simulink model "optper"  (Simulink 3.00)
settings: Solver=ode45  SolverMode=SingleTasking  StartTime=0.0  StopTime=250  RelTol=1e-5  AbsTol=1e-5
libraries: simulink_extras x1
settings Model: SaveTime=off  SaveOutput=off  RTWTemplateMakefile=grt_vc.tmf  LastModifiedBy=abonyij

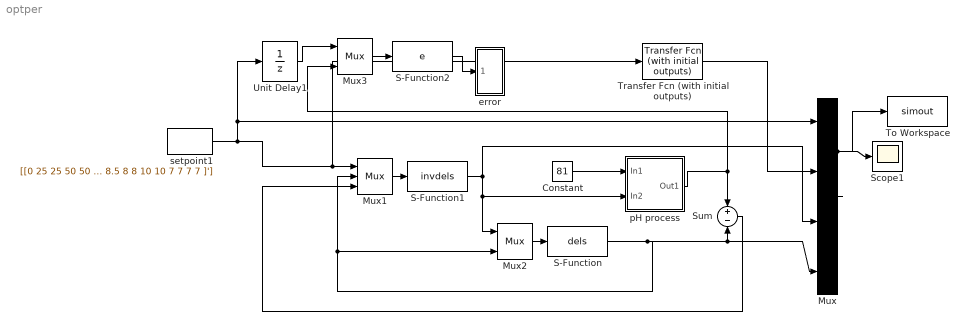
== system optper ==
  Constant : Constant  Value=81
  Mux : Mux  Inputs=4
      settings: DisplayOption=none
  Mux1 : Mux  Inputs=3
      settings: DisplayOption=none
  Mux2 : Mux  Inputs=2
      settings: DisplayOption=none
  Mux3 : Mux  Inputs=2
      settings: DisplayOption=none
  S-Function : S-Function  FunctionName=dels  PortCounts=[]  SFunctionModules=''
  S-Function1 : S-Function  FunctionName=invdels  PortCounts=[]  SFunctionModules=''
  S-Function2 : S-Function  FunctionName=e  PortCounts=[]  SFunctionModules=''
  Scope1 : Scope
      settings: TickLabels=on  TimeRange=auto  YMin=6  YMax=12  SaveName=pi  DataFormat=Matrix  SampleInput=on
  Sum : Sum  Inputs=+|-  SaturateOnIntegerOverflow=on
  To Workspace : ToWorkspace  VariableName=simout  SampleTime=0.2  SaveFormat=Matrix
  Transfer Fcn (with initial outputs) : simulink_extras/Additional Linear/Transfer Fcn (with initial outputs)  N=[1]  D=[0.2 1]  Y0=7  U0=7
  Unit Delay1 : UnitDelay  X0=7  SampleTime=0.2
  error : Subsystem
      mask Display: disp('IAE')
  pH process : Subsystem
  setpoint1 : FromWorkspace  VariableName=[[0 25 25 50 50 75 75 100 100 125 125 150 150 175 175 200 200 225 225 250 250]', [7 8 8 9 9 8 8 9.5 9.4 7.5 7.5 8.5 8.5 8 8 10 10 7 7 7 7 ]']  SampleTime=25  HoldFinalValue=on
  wires:
  Mux/1 -> Scope1/1, To Workspace/1
  Constant/1 -> pH process/1(In1)
  Mux2/1 -> S-Function/1
  Mux1/1 -> S-Function1/1
  S-Function1/1 -> Mux/3, pH process/2(In2), Mux2/1
  S-Function/1 -> Mux/4, Sum/2, Mux1/2, Mux2/2
  Sum/1 -> Mux1/3
  setpoint1/1 -> Mux/1, Unit Delay1/1, Mux1/1, Transfer Fcn (with initial outputs)/1
  S-Function2/1 -> error/1(in_1)
  Mux3/1 -> S-Function2/1
  Unit Delay1/1 -> Mux3/1
  pH process/1(Out1) -> Sum/1, Mux3/2
  Transfer Fcn (with initial outputs)/1 -> Mux/2

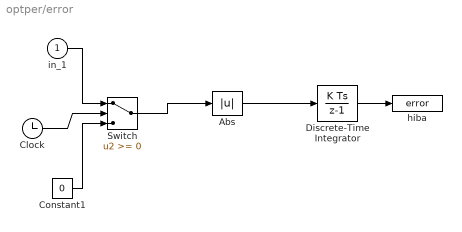
== system optper/error ==
  in_1 : Inport  Port=1  PortWidth=-1  SampleTime=-1  DataType=auto
      settings: SignalType=auto
  Abs : Abs
  Clock : Clock
      settings: DisplayTime=off  Decimation=10
  Constant1 : Constant  Value=0
  Discrete-Time Integrator : DiscreteIntegrator  IntegratorMethod=ForwardEuler  ExternalReset=none  InitialConditionSource=internal  InitialCondition=0  LimitOutput=off  UpperSaturationLimit=inf  LowerSaturationLimit=-inf  ShowSaturationPort=off  ShowStatePort=off  SampleTime=0.2
  Switch : Switch  Threshold=0
  hiba : ToWorkspace  VariableName=error  SampleTime=0  SaveFormat=Matrix
      settings: Buffer=1
  wires:
  Switch/1 -> Abs/1
  in_1/1 -> Switch/1
  Constant1/1 -> Switch/3
  Clock/1 -> Switch/2
  Abs/1 -> Discrete-Time Integrator/1
  Discrete-Time Integrator/1 -> hiba/1

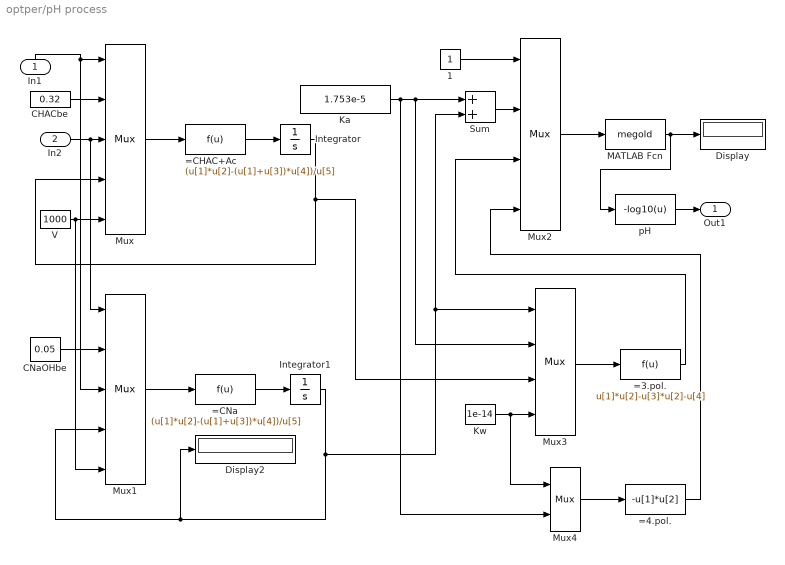
== system optper/pH process ==
  In1 : Inport  Orientation=up  Port=1  PortWidth=-1  SampleTime=-1  DataType=auto
      settings: SignalType=auto
  In2 : Inport  Port=2  PortWidth=-1  SampleTime=-1  DataType=auto
      settings: SignalType=auto
  1 : Constant  Value=1
  =3.pol. : Fcn  Expr=u[1]*u[2]-u[3]*u[2]-u[4]
  =4.pol. : Fcn  Expr=-u[1]*u[2]
  =CHAC+Ac : Fcn  Expr=(u[1]*u[2]-(u[1]+u[3])*u[4])/u[5]
  =CNa : Fcn  Expr=(u[1]*u[2]-(u[1]+u[3])*u[4])/u[5]
  CHACbe : Constant  Value=0.32
  CNaOHbe : Constant  Value=0.05
  Display : Display
      settings: Format=short
  Display2 : Display
      settings: Format=short
  Integrator : Integrator  ExternalReset=none  InitialConditionSource=internal  InitialCondition=0.0435  LimitOutput=off  UpperSaturationLimit=inf  LowerSaturationLimit=-inf  ShowSaturationPort=off  ShowStatePort=off  AbsoluteTolerance=auto
  Integrator1 : Integrator  ExternalReset=none  InitialConditionSource=internal  InitialCondition=0.0432  LimitOutput=off  UpperSaturationLimit=inf  LowerSaturationLimit=-inf  ShowSaturationPort=off  ShowStatePort=off  AbsoluteTolerance=auto
  Ka : Constant  Value=1.753e-5
  Kw : Constant  Value=1e-14
  MATLAB Fcn : MATLABFcn  MATLABFcn=megold  OutputWidth=1  OutputSignalType=auto
  Mux : Mux  Inputs=5
      settings: DisplayOption=none
  Mux1 : Mux  Inputs=5
      settings: DisplayOption=none
  Mux2 : Mux  Inputs=4
      settings: DisplayOption=none
  Mux3 : Mux  Inputs=4
      settings: DisplayOption=none
  Mux4 : Mux  Inputs=2
      settings: DisplayOption=none
  Sum : Sum  Inputs=++  SaturateOnIntegerOverflow=on
  V : Constant  Value=1000
  pH : Fcn  Expr=-log10(u)
  Out1 : Outport  Port=1  InitialOutput=0
  wires:
  CHACbe/1 -> Mux/2
  Mux/1 -> =CHAC+Ac/1
  =CHAC+Ac/1 -> Integrator/1
  In2/1 -> Mux/3, Mux1/1
  CNaOHbe/1 -> Mux1/2
  In1/1 -> Mux/1, Mux1/3
  =CNa/1 -> Integrator1/1
  Mux1/1 -> =CNa/1
  V/1 -> Mux/5, Mux1/5
  1/1 -> Mux2/1
  Integrator1/1 -> Display2/1, Mux1/4, Sum/2, Mux3/1
  Mux3/1 -> =3.pol./1
  Integrator/1 -> Mux/4, Mux3/3
  Mux4/1 -> =4.pol./1
  Kw/1 -> Mux3/4, Mux4/1
  Ka/1 -> Sum/1, Mux3/2, Mux4/2
  Sum/1 -> Mux2/2
  =3.pol./1 -> Mux2/3
  =4.pol./1 -> Mux2/4
  Mux2/1 -> MATLAB Fcn/1
  MATLAB Fcn/1 -> Display/1, pH/1
  pH/1 -> Out1/1
